simulink model "auv_modell_camsim_kalman2"  (Simulink 7.0)
settings: Solver=ode4  StartTime=0.0  StopTime=300  FixedStep=0.1  RelTol=1e-3
undefined symbols (not defined in the file or in its folder): ekf2
libraries: fordypningsprosjekt x3, simulink x1
settings Model: Creator=anderga  LastModifiedBy=anderga  ExtModeAutoUpdateStatusClock=off  BufferReuse=off
settings OptimizationCC: BlockReduction=off  InlineParams=on  BufferReuse=off

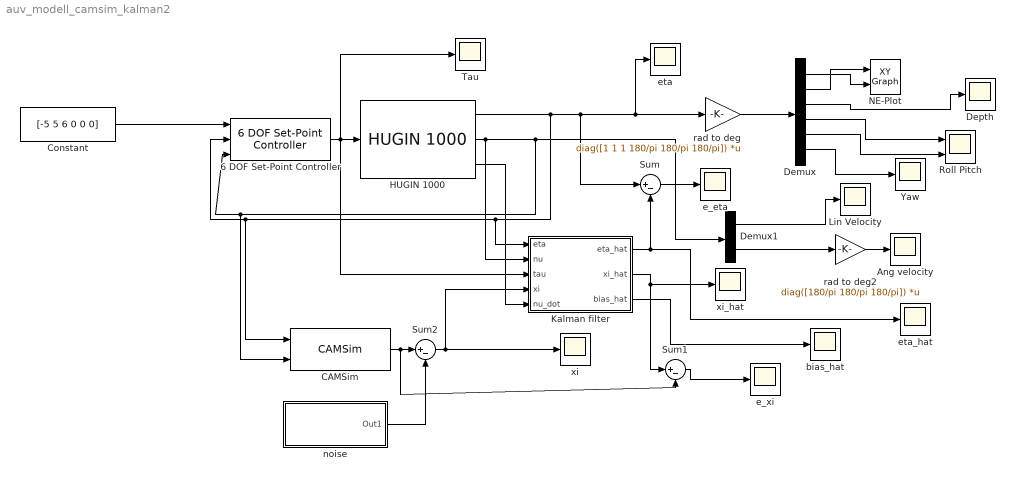
== system auv_modell_camsim_kalman2 ==
  6 DOF Set-Point Controller : fordypningsprosjekt/6 DOF Set-Point Controller  SystemSampleTime=-1  Kp=diag([230 300 1000])  Ki=diag([2 5 0])  Kd=diag([750 700 0])  depthPID=[50, 1, 0]  rollPID=[0, 0, 0]  pitchPID=[500, 2, 50]  sat=1000.*[1, 1, 1, 1, 1, 1]
  Ang velocity : Scope
      settings: YMin=-0.45  YMax=0.05  SaveName=ScopeData6
  CAMSim : fordypningsprosjekt/CAMSim  SystemSampleTime=-1  bottom=10
  Constant : Constant  Value=[-5 5 6 0 0 0]  OutDataType=sfix(16)  OutScaling=2^0
  Demux : Demux  Outputs=6
  Demux1 : Demux  Outputs=2
  Depth : Scope
      settings: TimeRange=400  YMin=-140  YMax=40  SaveName=ScopeData4
  HUGIN 1000 : fordypningsprosjekt/HUGIN 1000  SystemSampleTime=-1  eta_0=eta0  nu_0=[0 0 0 0 0 0]
  Kalman filter : Subsystem
  Lin Velocity : Scope
      settings: YMin=-3.46945e-018  YMax=0.1
  NE-Plot : simulink/Sinks/XY Graph  SystemSampleTime=-1  xmin=-100  xmax=220  ymin=-100  ymax=1000  st=-1
  Roll Pitch : Scope  NumInputPorts=2
      settings: TimeRange=400  YMin=-1~-1  YMax=1~1  SaveName=ScopeData3
  Sum : Sum  Inputs=|+-  OutDataType=sfix(16)  OutScaling=2^0
  Sum1 : Sum  Inputs=|+-  OutDataType=sfix(16)  OutScaling=2^0
  Sum2 : Sum  Inputs=|+-  OutDataType=sfix(16)  OutScaling=2^0
  Tau : Scope
      settings: TimeRange=100  YMin=-0.005  YMax=0.0225
  Yaw : Scope
      settings: TimeRange=100  YMin=-1  YMax=1  SaveName=ScopeData2
  bias_hat : Scope
      settings: YMin=-25  YMax=200  SaveName=ScopeData11
  e_eta : Scope
      settings: YMin=-25  YMax=2.5  SaveName=ScopeData14
  e_xi : Scope
      settings: YMin=-6  YMax=4  SaveName=ScopeData15
  eta : Scope
      settings: YMin=-10  YMax=7.5  SaveName=ScopeData7
  eta_hat : Scope
      settings: YMin=-10  YMax=30  SaveName=ScopeData9
  noise : Subsystem
  rad to deg : Gain  Gain=diag([1 1 1 180/pi 180/pi 180/pi])  Multiplication=Matrix(K*u)  ParameterDataType=sfix(16)  ParameterScaling=2^0  OutDataType=sfix(16)  OutScaling=2^0
  rad to deg2 : Gain  Gain=diag([180/pi 180/pi 180/pi])  Multiplication=Matrix(K*u)  ParameterDataType=sfix(16)  ParameterScaling=2^0  OutDataType=sfix(16)  OutScaling=2^0
  xi : Scope
      settings: TimeRange=100  YMin=-7  YMax=7  SaveName=ScopeData13
  xi_hat : Scope
      settings: TimeRange=100  YMin=-7  YMax=7  SaveName=ScopeData5
  wires:
  HUGIN 1000/1 -> Sum/1, rad to deg/1, eta/1, Kalman filter/1(eta), 6 DOF Set-Point Controller/2, CAMSim/1
  Demux/2 -> NE-Plot/1
  Demux/1 -> NE-Plot/2
  Demux/6 -> Yaw/1
  Demux/4 -> Roll Pitch/1
  Demux/5 -> Roll Pitch/2
  Demux/3 -> Depth/1
  Demux1/1 -> Lin Velocity/1
  Demux1/2 -> rad to deg2/1
  HUGIN 1000/2 -> CAMSim/2, 6 DOF Set-Point Controller/3, Demux1/1, Kalman filter/2(nu)
  rad to deg/1 -> Demux/1
  rad to deg2/1 -> Ang velocity/1
  Kalman filter/1(eta_hat) -> eta_hat/1, Sum/2
  Kalman filter/3(bias_hat) -> bias_hat/1
  Sum/1 -> e_eta/1
  Sum1/1 -> e_xi/1
  CAMSim/1 -> Sum2/1, Sum1/2
  noise/1(Out1) -> Sum2/2
  Sum2/1 -> xi/1, Kalman filter/4(xi)
  6 DOF Set-Point Controller/1 -> Tau/1, HUGIN 1000/1, Kalman filter/3(tau)
  Constant/1 -> 6 DOF Set-Point Controller/1
  HUGIN 1000/3 -> Kalman filter/5(nu_dot)
  Kalman filter/2(xi_hat) -> Sum1/1, xi_hat/1

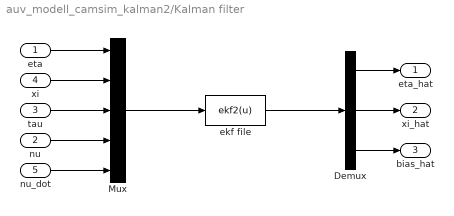
== system auv_modell_camsim_kalman2/Kalman filter ==
  eta : Inport  OutDataType=sfix(16)  OutScaling=2^0
  nu : Inport  Port=2  OutDataType=sfix(16)  OutScaling=2^0
  tau : Inport  Port=3  OutDataType=sfix(16)  OutScaling=2^0
  xi : Inport  Port=4  OutDataType=sfix(16)  OutScaling=2^0
  nu_dot : Inport  Port=5  OutDataType=sfix(16)  OutScaling=2^0
  Demux : Demux  Outputs=3
  Mux : Mux  Inputs=5
  ekf file : MATLABFcn  MATLABFcn=ekf2(u)  OutputDimensions=18
  eta_hat : Outport  OutDataType=sfix(16)  OutScaling=2^0
  xi_hat : Outport  Port=2  OutDataType=sfix(16)  OutScaling=2^0
  bias_hat : Outport  Port=3  OutDataType=sfix(16)  OutScaling=2^0
  wires:
  eta/1 -> Mux/1
  Demux/1 -> eta_hat/1
  Demux/2 -> xi_hat/1
  Demux/3 -> bias_hat/1
  Mux/1 -> ekf file/1
  ekf file/1 -> Demux/1
  xi/1 -> Mux/2
  tau/1 -> Mux/3
  nu/1 -> Mux/4
  nu_dot/1 -> Mux/5

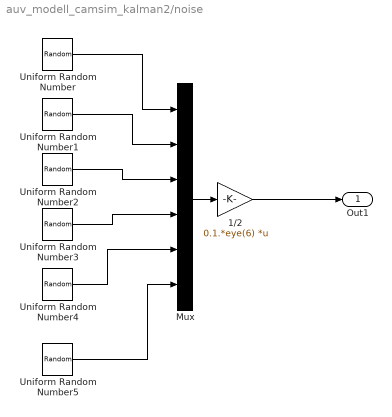
== system auv_modell_camsim_kalman2/noise ==
  1/2 : Gain  Gain=0.1.*eye(6)  Multiplication=Matrix(K*u)  ParameterDataType=sfix(16)  ParameterScaling=2^0  OutDataType=sfix(16)  OutScaling=2^0
  Mux : Mux  Inputs=6
  Uniform Random Number : UniformRandomNumber  Seed=15  SampleTime=0
  Uniform Random Number1 : UniformRandomNumber  Seed=16  SampleTime=0
  Uniform Random Number2 : UniformRandomNumber  Seed=17  SampleTime=0
  Uniform Random Number3 : UniformRandomNumber  Seed=18  SampleTime=0
  Uniform Random Number4 : UniformRandomNumber  Seed=19  SampleTime=0
  Uniform Random Number5 : UniformRandomNumber  Seed=20  SampleTime=0
  Out1 : Outport  OutDataType=sfix(16)  OutScaling=2^0
  wires:
  Mux/1 -> 1/2/1
  Uniform Random Number5/1 -> Mux/6
  Uniform Random Number4/1 -> Mux/5
  Uniform Random Number3/1 -> Mux/4
  Uniform Random Number2/1 -> Mux/3
  Uniform Random Number1/1 -> Mux/2
  Uniform Random Number/1 -> Mux/1
  1/2/1 -> Out1/1
